simulink model "LIN_F16Block_lo"  (Simulink 9.2)
settings: Solver=ode5  StartTime=0.0  StopTime=20  FixedStep=0.001  RelTol=1e-3  EnableMultiTasking=on
model workspace (MAT data in the model file):
  x_a : num (value not decoded)
values from neighbouring files (symbols this model uses):
  dLEF = xu(17)    [trim_F16.m]    (also in trim_steady_state.m; trimfun.m = 0)
  fi_flag_Simulink = 0    [FindF16Dynamics.m]    (also in normal_response_wrt_acc_pos.m; runF16Sim.m = 1; runLINF16sim.m; sim_F16_lo.m)
  trim_control = trim_control_lo    [runLINF16sim.m]    (also in trim_F16.m = [UX(2);UX(4);UX(5)]; trim_steady_state.m = [UX(2);UX(4);UX(5)])
  trim_state = xu_lo    [runLINF16sim.m]    (also in trim_F16.m = xu(1:12); trim_steady_state.m = xu(1:12))
  trim_state_lin = trim_state_lo    [FindF16Dynamics.m]    (also in runLINF16sim.m; terrain_following_model.m = [trim.trim_state_lo; trim.thrust; trim.trim_control_lo])
  trim_thrust = trim_thrust_lo    [runLINF16sim.m]    (also in trim_F16.m = UX(1); trim_steady_state.m = UX(1))
  x_a = 0    [accelerometer.m]
settings Model: LogicAnalyzerSignalOrdering=3751009d-1ef9-4209-ac4d-0382ac61319a,47dae349-736d-4eb0-a341-24b18976b090,3f464a83-68a8-4c86-8a43-d5bdbd0606c4,26ebb13d-b3a3-4491-8361-bfc3f4fc3115,ef2fde50-04bd-4c56-89ff-2e03a98dcbde  Creator=keviczky  LastModifiedBy=lorenzoterenzi  ExtModeAutoUpdateStatusClock=off
settings DataIOCC: Decimation=50  ExternalInput=[0 2120.62144781519 -2.46068617229406 2.91286693086823e-16 2.79661206579015e-15]  InitialState=[]  LimitDataPoints=off  LoadExternalInput=on  LoadInitialState=on  SignalLoggingSaveFormat=Dataset  SignalLoggingName=sigsOut
settings OptimizationCC: BooleanDataType=off  DefaultParameterBehavior=Inlined  BufferReuse=off  LifeSpan=auto
settings DebuggingCC: SaveWithParameterizedLinksMsg=none  SignalResolutionControl=TryResolveAllWithWarning  MultiTaskDSMMsg=warning  MultiTaskCondExecSysMsg=none  FcnCallInpInsideContextMsg=error  StateNameClashWarn=none  InitInArrayFormatMsg=none  SFUnexpectedBacktrackingDiag=error  SFNoUnconditionalDefaultTransitionDiag=error  SFExecutionAtInitializationDiag=warning
settings HardwareCC: TargetUnknown=on
settings SFSimCC: SimUseLocalCustomCode=on
settings RTWCC: RTWUseLocalCustomCode=on
settings CodeAppCC: StateflowObjectComments=off
settings GRTTargetCC: TargetLangStandard=C99 (ISO)  GeneratePreprocessorConditionals=Use local settings
settings ConfigComp: CovExternalEMLEnable=on

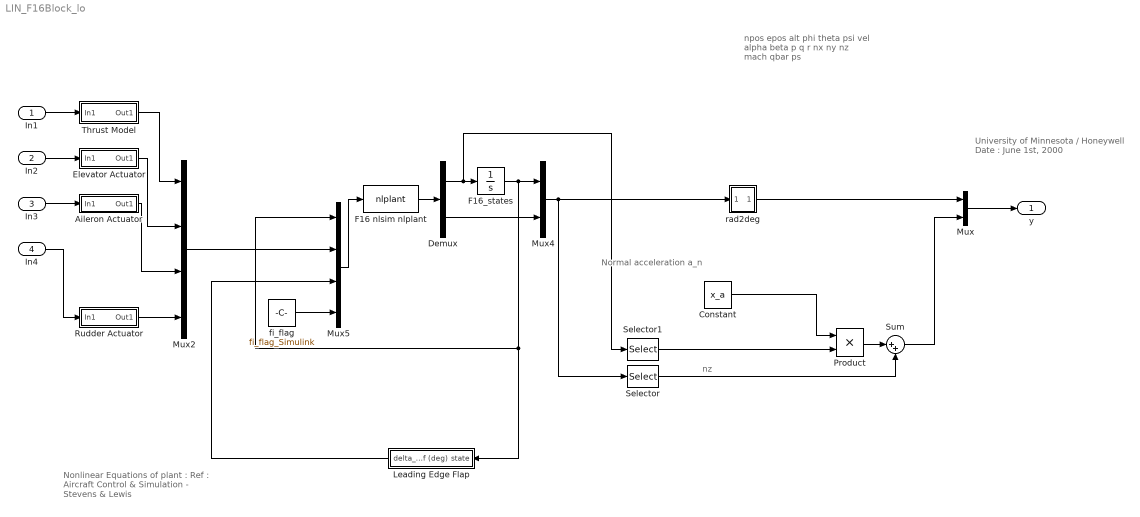
== system LIN_F16Block_lo ==
  note: Normal acceleration a_n
  note: npos
      | epos
      | alt
      | phi
      | theta
      | psi
      | vel
      | alpha
      | beta
      | p
      | q
      | r
      | nx
      | ny
      | nz
      | mach
      | qbar
      | ps
  note: University of Minnesota / Honeywell
      | Date : June 1st, 2000
  note: Nonlinear Equations of plant :
      | Ref : Aircraft Control & Simulation
      | - Stevens & Lewis
  note: nz
  In1 : Inport
  In2 : Inport  Port=2
  In3 : Inport  Port=3
  In4 : Inport  Port=4
  Aileron Actuator : Subsystem  AncestorBlock=F16_Actuator_Library/Aileron Actuator
  Constant : Constant  Value=x_a
  Demux : Demux  Outputs=[12 6]
  Elevator Actuator : Subsystem  AncestorBlock=F16_Actuator_Library/Elevator Actuator
  F16 nlsim nlplant : MATLABFcn  MATLABFcn=nlplant  OutputDimensions=18  OutputSignalType=real
  F16_states : Integrator  InitialCondition=trim_state
  Leading Edge Flap : Subsystem
  Mux : Mux  Inputs=2
  Mux2 : Mux
  Mux4 : Mux  Inputs=2
  Mux5 : Mux  Inputs=[12 4 1 1]
  Product : Product
  Rudder Actuator : Subsystem  AncestorBlock=F16_Actuator_Library/Rudder Actuator
  Selector : Selector  InputPortWidth=18  IndexOptions=Index vector (dialog)  Indices=[15]  OutputSizes=1
  Selector1 : Selector  InputPortWidth=12  IndexOptions=Index vector (dialog)  Indices=[11]  OutputSizes=1
  Sum : Sum  Inputs=|++
  Thrust Model : Subsystem  AncestorBlock=F16_Actuator_Library/Thrust Model
  fi_flag : Constant  Value=fi_flag_Simulink
  rad2deg : Subsystem
  y : Outport
  wires:
  F16 nlsim nlplant/1 -> Demux/1
  Demux/1 -> Selector1/1, F16_states/1
  Demux/2 -> Mux4/2
  Mux5/1 -> F16 nlsim nlplant/1
  Mux2/1 -> Mux5/2
  F16_states/1 -> Mux5/1, Leading Edge Flap/1(state), Mux4/1
  In1/1 -> Thrust Model/1(In1)
  In2/1 -> Elevator Actuator/1(In1)
  In3/1 -> Aileron Actuator/1(In1)
  In4/1 -> Rudder Actuator/1(In1)
  fi_flag/1 -> Mux5/4
  Leading Edge Flap/1(delta_lef (deg)) -> Mux5/3
  Elevator Actuator/1(Out1) -> Mux2/2
  Aileron Actuator/1(Out1) -> Mux2/3
  Rudder Actuator/1(Out1) -> Mux2/4
  Thrust Model/1(Out1) -> Mux2/1
  rad2deg/1(Out1) -> Mux/1
  Sum/1 -> Mux/2
  Mux/1 -> y/1
  Constant/1 -> Product/1
  Selector1/1 -> Product/2
  Product/1 -> Sum/1
  Mux4/1 -> Selector/1, rad2deg/1(In1)
  Selector/1 -> Sum/2

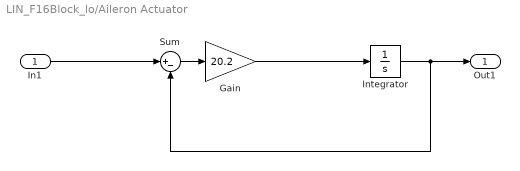
== system LIN_F16Block_lo/Aileron Actuator ==
  In1 : Inport
  Gain : Gain  Gain=20.2  SaturateOnIntegerOverflow=on  OutDataTypeStr=Inherit: Same as input  ParamDataTypeStr=Inherit: Same as input
  "Integrator " : Integrator  InitialCondition=trim_control(2)  UpperSaturationLimit=21.5  LowerSaturationLimit=-21.5
  Sum : Sum  Inputs=|+-  SaturateOnIntegerOverflow=on  InputSameDT=on  OutDataTypeStr=Inherit: Same as first input
  Out1 : Outport
  wires:
  "Integrator "/1 -> Sum/2, Out1/1
  Gain/1 -> "Integrator "/1
  Sum/1 -> Gain/1
  In1/1 -> Sum/1

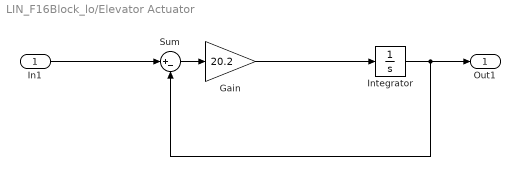
== system LIN_F16Block_lo/Elevator Actuator ==
  In1 : Inport
  Gain : Gain  Gain=20.2  SaturateOnIntegerOverflow=on  OutDataTypeStr=Inherit: Same as input  ParamDataTypeStr=Inherit: Same as input
  "Integrator " : Integrator  InitialCondition=trim_control(1)  UpperSaturationLimit=25  LowerSaturationLimit=-25
  Sum : Sum  Inputs=|+-  SaturateOnIntegerOverflow=on  InputSameDT=on  OutDataTypeStr=Inherit: Same as first input
  Out1 : Outport
  wires:
  "Integrator "/1 -> Sum/2, Out1/1
  Gain/1 -> "Integrator "/1
  Sum/1 -> Gain/1
  In1/1 -> Sum/1

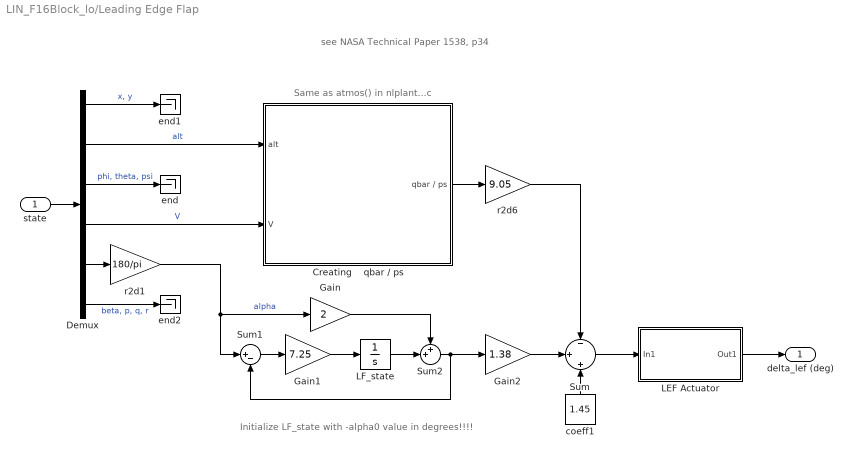
== system LIN_F16Block_lo/Leading Edge Flap ==
  note: see NASA Technical Paper 1538, p34
  note: Same as atmos() in nlplant...c
  note: Initialize LF_state with -alpha0 value in degrees!!!!
  state : Inport
  Creating    qbar / ps : Subsystem
  Demux : Demux  Outputs=[2,1,3,1,1,4]
  Gain : Gain  Gain=2  SaturateOnIntegerOverflow=on  OutDataTypeStr=Inherit: Same as input  ParamDataTypeStr=Inherit: Same as input
  Gain1 : Gain  Gain=7.25  SaturateOnIntegerOverflow=on  OutDataTypeStr=Inherit: Same as input  ParamDataTypeStr=Inherit: Same as input
  Gain2 : Gain  Gain=1.38  SaturateOnIntegerOverflow=on  OutDataTypeStr=Inherit: Same as input  ParamDataTypeStr=Inherit: Same as input
  LEF Actuator : Subsystem  AncestorBlock=F16_Actuator_Library/Aileron Actuator
  LF_state : Integrator  InitialCondition=-trim_state_lin(8)*180/pi
  Sum : Sum  Inputs=-|+|+  SaturateOnIntegerOverflow=on  InputSameDT=on  OutDataTypeStr=Inherit: Same as first input
  Sum1 : Sum  Inputs=|+-  SaturateOnIntegerOverflow=on  InputSameDT=on  OutDataTypeStr=Inherit: Same as first input
  Sum2 : Sum  Inputs=++|  SaturateOnIntegerOverflow=on  InputSameDT=on  OutDataTypeStr=Inherit: Same as first input
  coeff1 : Constant  Value=1.45
  end : Terminator
  end1 : Terminator
  end2 : Terminator
  r2d1 : Gain  Gain=180/pi  SaturateOnIntegerOverflow=on  OutDataTypeStr=Inherit: Same as input  ParamDataTypeStr=Inherit: Same as input
  r2d6 : Gain  Gain=9.05  SaturateOnIntegerOverflow=on  OutDataTypeStr=Inherit: Same as input  ParamDataTypeStr=Inherit: Same as input
  delta_lef (deg) : Outport
  wires:
  LEF Actuator/1(Out1) -> delta_lef (deg)/1
  Sum/1 -> LEF Actuator/1(In1)
  Demux/3 -> end/1  "phi, theta, psi"
  state/1 -> Demux/1
  Sum1/1 -> Gain1/1
  Gain1/1 -> LF_state/1
  Gain/1 -> Sum2/1
  Gain2/1 -> Sum/2
  Demux/1 -> end1/1  "x, y"
  Demux/5 -> r2d1/1
  Demux/6 -> end2/1  "beta, p, q, r"
  coeff1/1 -> Sum/3
  Sum2/1 -> Sum1/2, Gain2/1
  LF_state/1 -> Sum2/2
  r2d1/1 -> Sum1/1, Gain/1  "alpha"
  Demux/4 -> Creating    qbar / ps/2(V)  "V"
  Creating    qbar / ps/1(qbar / ps) -> r2d6/1
  r2d6/1 -> Sum/1
  Demux/2 -> Creating    qbar / ps/1(alt)  "alt"

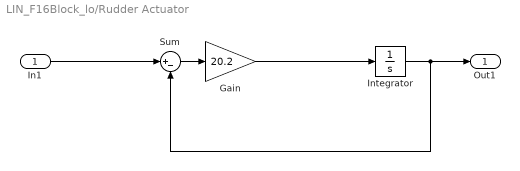
== system LIN_F16Block_lo/Rudder Actuator ==
  In1 : Inport
  Gain : Gain  Gain=20.2  SaturateOnIntegerOverflow=on  OutDataTypeStr=Inherit: Same as input  ParamDataTypeStr=Inherit: Same as input
  "Integrator " : Integrator  InitialCondition=trim_control(3)  UpperSaturationLimit=30  LowerSaturationLimit=-30
  Sum : Sum  Inputs=|+-  SaturateOnIntegerOverflow=on  InputSameDT=on  OutDataTypeStr=Inherit: Same as first input
  Out1 : Outport
  wires:
  "Integrator "/1 -> Sum/2, Out1/1
  Gain/1 -> "Integrator "/1
  Sum/1 -> Gain/1
  In1/1 -> Sum/1

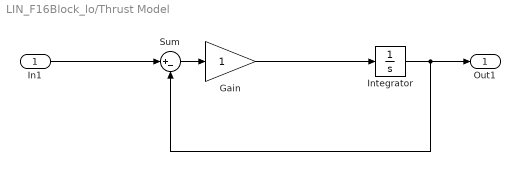
== system LIN_F16Block_lo/Thrust Model ==
  In1 : Inport
  Gain : Gain  SaturateOnIntegerOverflow=on  OutDataTypeStr=Inherit: Same as input  ParamDataTypeStr=Inherit: Same as input
  "Integrator " : Integrator  InitialCondition=trim_thrust  UpperSaturationLimit=30  LowerSaturationLimit=-30
  Sum : Sum  Inputs=|+-  SaturateOnIntegerOverflow=on  InputSameDT=on  OutDataTypeStr=Inherit: Same as first input
  Out1 : Outport
  wires:
  "Integrator "/1 -> Sum/2, Out1/1
  Gain/1 -> "Integrator "/1
  Sum/1 -> Gain/1
  In1/1 -> Sum/1

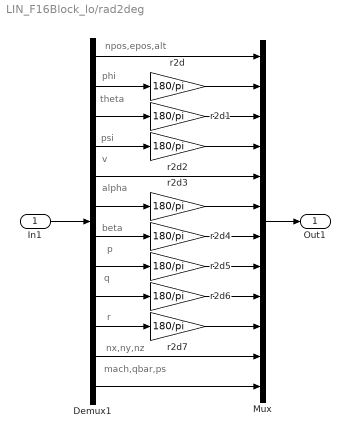
== system LIN_F16Block_lo/rad2deg ==
  note: npos,epos,alt
  note: phi
  note: theta
  note: psi
  note: v
  note: alpha
  note: beta
  note: p
  note: q
  note: r
  note: nx,ny,nz
  note: mach,qbar,ps
  In1 : Inport
  Demux1 : Demux  Outputs=[3 1 1 1 1 1 1 1 1 1 3 3]
  Mux : Mux  Inputs=[3 1 1 1 1 1 1 1 1 1 3 3]
  r2d{,1..7} (8 alike) : Gain  Gain=180/pi  SaturateOnIntegerOverflow=on  OutDataTypeStr=Inherit: Same as input  ParamDataTypeStr=Inherit: Same as input
  Out1 : Outport
  wires:
  In1/1 -> Demux1/1
  Demux1/2 -> r2d/1
  Demux1/3 -> r2d1/1
  Demux1/4 -> r2d2/1
  Demux1/1 -> Mux/1
  Demux1/5 -> Mux/5
  r2d2/1 -> Mux/4
  r2d1/1 -> Mux/3
  r2d/1 -> Mux/2
  Demux1/6 -> r2d3/1
  Demux1/7 -> r2d4/1
  Demux1/8 -> r2d5/1
  Demux1/9 -> r2d6/1
  Demux1/10 -> r2d7/1
  r2d3/1 -> Mux/6
  r2d4/1 -> Mux/7
  r2d5/1 -> Mux/8
  r2d6/1 -> Mux/9
  r2d7/1 -> Mux/10
  Mux/1 -> Out1/1
  Demux1/11 -> Mux/11
  Demux1/12 -> Mux/12

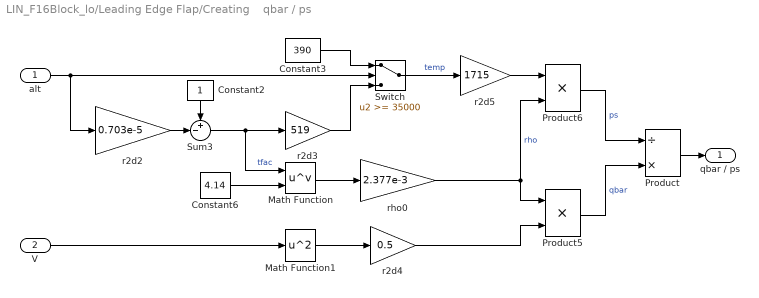
== system LIN_F16Block_lo/Leading Edge Flap/Creating    qbar / ps ==
  alt : Inport
  V : Inport  Port=2
  Constant2 : Constant
  Constant3 : Constant  Value=390
  Constant6 : Constant  Value=4.14
  Math Function : Math  Operator=pow  SaturateOnIntegerOverflow=on
  Math Function1 : Math  Operator=square  SaturateOnIntegerOverflow=on
  Product : Product  Inputs=/*  SaturateOnIntegerOverflow=on  InputSameDT=on  OutDataTypeStr=Inherit: Same as first input
  Product5 : Product  Inputs=**  SaturateOnIntegerOverflow=on  InputSameDT=on  OutDataTypeStr=Inherit: Same as first input
  Product6 : Product  Inputs=**  SaturateOnIntegerOverflow=on  InputSameDT=on  OutDataTypeStr=Inherit: Same as first input
  Sum3 : Sum  Inputs=+-|  SaturateOnIntegerOverflow=on  InputSameDT=on  OutDataTypeStr=Inherit: Same as first input
  Switch : Switch  Threshold=35000  SaturateOnIntegerOverflow=on  InputSameDT=on
  r2d2 : Gain  Gain=0.703e-5  SaturateOnIntegerOverflow=on  OutDataTypeStr=Inherit: Same as input  ParamDataTypeStr=Inherit: Same as input
  r2d3 : Gain  Gain=519  SaturateOnIntegerOverflow=on  OutDataTypeStr=Inherit: Same as input  ParamDataTypeStr=Inherit: Same as input
  r2d4 : Gain  Gain=0.5  SaturateOnIntegerOverflow=on  OutDataTypeStr=Inherit: Same as input  ParamDataTypeStr=Inherit: Same as input
  r2d5 : Gain  Gain=1715  SaturateOnIntegerOverflow=on  OutDataTypeStr=Inherit: Same as input  ParamDataTypeStr=Inherit: Same as input
  rho0 : Gain  Gain=2.377e-3  SaturateOnIntegerOverflow=on  OutDataTypeStr=Inherit: Same as input  ParamDataTypeStr=Inherit: Same as input
  qbar / ps : Outport
  wires:
  alt/1 -> r2d2/1, Switch/2
  Sum3/1 -> Math Function/1, r2d3/1  "tfac"
  Constant3/1 -> Switch/1
  r2d3/1 -> Switch/3
  Constant6/1 -> Math Function/2
  rho0/1 -> Product5/1, Product6/2  "rho"
  Math Function1/1 -> r2d4/1
  r2d2/1 -> Sum3/2
  Constant2/1 -> Sum3/1
  Math Function/1 -> rho0/1
  r2d4/1 -> Product5/2
  Switch/1 -> r2d5/1  "temp"
  r2d5/1 -> Product6/1
  Product6/1 -> Product/1  "ps"
  Product5/1 -> Product/2  "qbar"
  Product/1 -> qbar / ps/1
  V/1 -> Math Function1/1

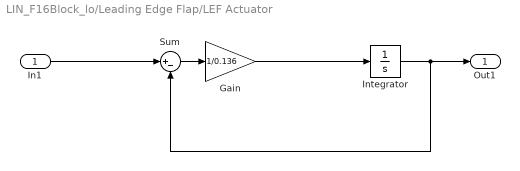
== system LIN_F16Block_lo/Leading Edge Flap/LEF Actuator ==
  In1 : Inport
  Gain : Gain  Gain=1/0.136  SaturateOnIntegerOverflow=on  OutDataTypeStr=Inherit: Same as input  ParamDataTypeStr=Inherit: Same as input
  "Integrator " : Integrator  InitialCondition=dLEF  UpperSaturationLimit=21.5  LowerSaturationLimit=-21.5
  Sum : Sum  Inputs=|+-  SaturateOnIntegerOverflow=on  InputSameDT=on  OutDataTypeStr=Inherit: Same as first input
  Out1 : Outport
  wires:
  "Integrator "/1 -> Sum/2, Out1/1
  Gain/1 -> "Integrator "/1
  Sum/1 -> Gain/1
  In1/1 -> Sum/1
